simulink subsystem "SystemInputsSimFocQep"  (R2024a)
settings: Solver=VariableStepAuto  StartTime=0.0  StopTime=10.0  RelTol=1e-3
undefined symbols (not defined in the file or in its folder): pmsm
libraries: simulink x1
settings Model: Creator=The MathWorks, Inc.  LastModifiedBy=I52209
settings RTWCC: GPUComputeCapability=3.5

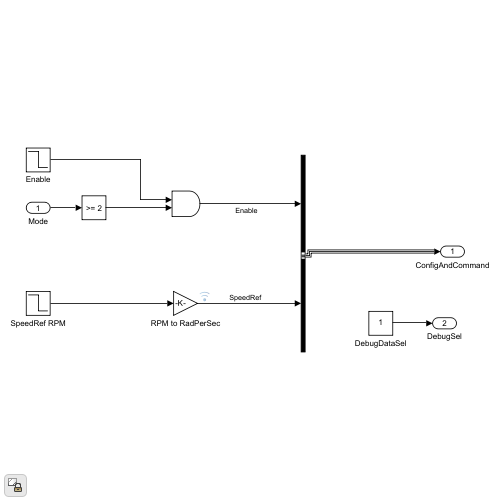
[thumbnail: Simulink's stored preview of the top-level diagram]
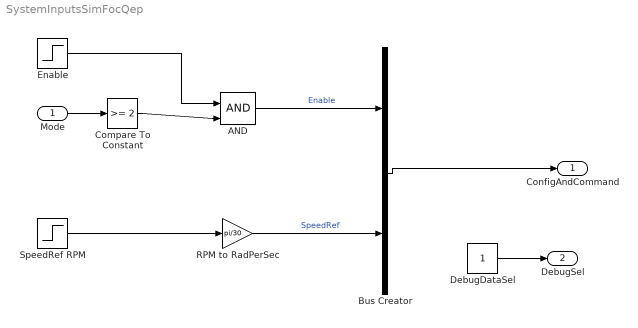
== system SystemInputsSimFocQep ==
  Mode : Inport
  AND : Logic  IconShape=distinctive  AllPortsSameDT=off  OutDataTypeStr=boolean
  Bus Creator : BusCreator  Inputs=2
  Compare To Constant : simulink/Logic and Bit Operations/Compare To Constant  relop=>=  const=2  OutDataTypeStr=boolean
  DebugDataSel : Constant  OutDataTypeStr=uint8  SampleTime=-1
  Enable : Step  Time=9.5  Before=1  After=0  OutDataTypeStr=dataType
  RPM to RadPerSec : Gain  Gain=pi/30  RndMeth=Simplest  OutDataTypeStr=Inherit: Same as input
  SpeedRef RPM : Step  Time=6  Before=pmsm.N_base * 0.5  After=-pmsm.N_base * 0.5  OutDataTypeStr=dataType
  ConfigAndCommand : Outport
  DebugSel : Outport  Port=2
  wires:
  DebugDataSel/1 -> DebugSel/1
  RPM to RadPerSec/1 -> Bus Creator/2  "SpeedRef"
  Enable/1 -> AND/1
  AND/1 -> Bus Creator/1  "Enable"
  Mode/1 -> Compare To Constant/1
  Bus Creator/1 -> ConfigAndCommand/1
  SpeedRef RPM/1 -> RPM to RadPerSec/1
  Compare To Constant/1 -> AND/2
